simulink model "planLocalPathMPPI"  (R2024b)
settings: Solver=FixedStepAuto  StartTime=0.0  StopTime=inf  RelTol=1e-3  SampleTimeConstraint=STIndependent
StartFcn:
  | % clf
  | % rng(1,"twister");
  | % set_param([bdroot(gcb) '/TaskControllerIn/Simulink Signals/Confirm New Goal/newGoalBlock'],'Value','goalPose');
settings Model: Creator=cstabile  LastModifiedBy=apattass
settings DataIOCC: SaveOutput=off  SaveTime=off
settings OptimizationCC: BlockReduction=off  EnhancedBackFolding=on  PassReuseOutputArgsAs=Individual arguments  ZeroExternalMemoryAtStartup=off  ZeroInternalMemoryAtStartup=off  MaxStackSize=64  OptimizeBlockOrder=speed  DifferentSizesBufferReuse=on  OptimizationCustomize=off  EfficientTunableParamExpr=on
settings DebuggingCC: IntegerOverflowMsg=none  ParameterTunabilityLossMsg=error
settings ModelReferenceCC: UpdateModelReferenceTargets=IfOutOfDate
settings SFSimCC: SFSimEcho=off  SimTargetLang=C++
settings RTWCC: Description=Embedded Coder  SystemTargetFile=ert.tlc  TemplateMakefile=ert_default_tmf  Toolchain=Colcon Tools  GPUComputeCapability=3.5
settings CodeAppCC: ForceParamTrailComments=on  IgnoreCustomStorageClasses=off  OperatorAnnotations=on  SimulinkDataObjDesc=on  SFDataObjDesc=on  InsertBlockDesc=on
settings ERTTargetCC: InlinedParameterPlacement=Hierarchical  RootIOFormat=Structure reference  ERTCustomFileTemplate=example_file_process.tlc  DynamicArrayContainerType=coder::array

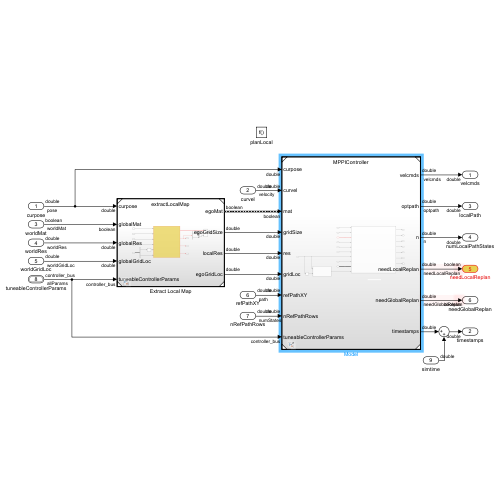
[thumbnail: Simulink's stored preview of the top-level diagram]
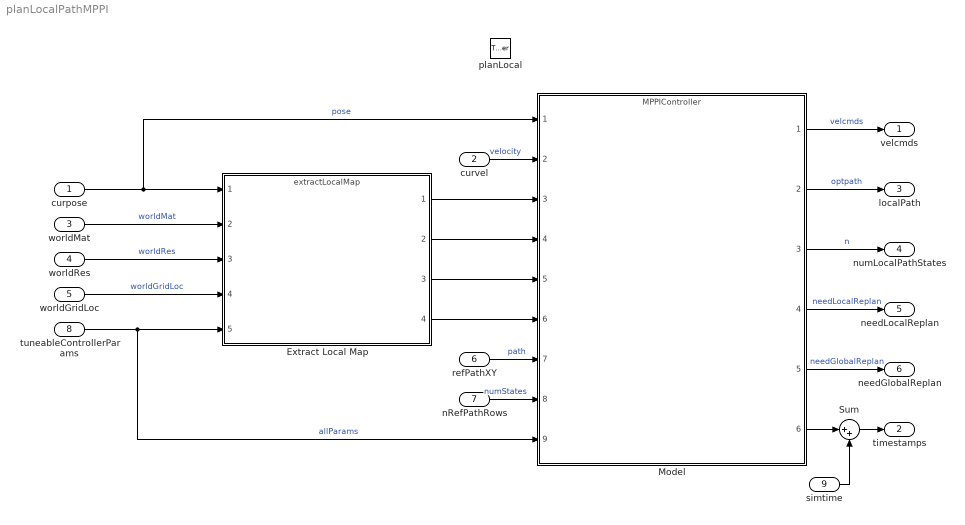
== system planLocalPathMPPI ==
  curpose : Inport  OutDataTypeStr=double  PortDimensions=3
  curvel : Inport  Port=2  OutDataTypeStr=double  PortDimensions=[1 2]
  worldMat : Inport  Port=3  OutDataTypeStr=boolean  PortDimensions=[1201 1201]
  worldRes : Inport  Port=4  OutDataTypeStr=double  PortDimensions=1
  worldGridLoc : Inport  Port=5  OutDataTypeStr=double  PortDimensions=2
  refPathXY : Inport  Port=6  OutDataTypeStr=double  PortDimensions=[10000 3]
  nRefPathRows : Inport  Port=7  OutDataTypeStr=double  PortDimensions=1
  tuneableControllerParams : Inport  Port=8  OutDataTypeStr=Bus: controller_bus  PortDimensions=1  BusOutputAsStruct=on
  simtime : Inport  Port=9  OutDataTypeStr=double  PortDimensions=1
  planLocal : TriggerPort  TriggerType=function-call  VariantControl=(inherit)  PortDimensions=1  TriggerSignalSampleTime=[0.10000000000000001,0]
  Extract Local Map : ModelReference  ModelNameDialog=extractLocalMap.slx  SimulationMode=Normal  ModelReferenceVersion=2.14
  Model : ModelReference  ModelNameDialog=MPPIController.slx  SimulationMode=Normal  ModelReferenceVersion=1.164
  Sum : Sum  Inputs=|++
  velcmds : Outport  OutDataTypeStr=double  PortDimensions=[1000 2]
  timestamps : Outport  Port=2  OutDataTypeStr=double  PortDimensions=[1000 1]
  localPath : Outport  Port=3  OutDataTypeStr=double  PortDimensions=[1000 3]
  numLocalPathStates : Outport  Port=4  OutDataTypeStr=double  PortDimensions=1
  needLocalReplan : Outport  Port=5  OutDataTypeStr=boolean  PortDimensions=1
  needGlobalReplan : Outport  Port=6  OutDataTypeStr=boolean  PortDimensions=1
  wires:
  curpose/1 -> Extract Local Map/1, Model/1  "pose"
  worldMat/1 -> Extract Local Map/2  "worldMat"
  tuneableControllerParams/1 -> Extract Local Map/5, Model/9  "allParams"
  worldRes/1 -> Extract Local Map/3  "worldRes"
  worldGridLoc/1 -> Extract Local Map/4  "worldGridLoc"
  nRefPathRows/1 -> Model/8  "numStates"
  Model/1 -> velcmds/1  "velcmds"
  Model/4 -> needLocalReplan/1  "needLocalReplan"
  Model/3 -> numLocalPathStates/1  "n"
  Model/2 -> localPath/1  "optpath"
  Model/5 -> needGlobalReplan/1  "needGlobalReplan"
  refPathXY/1 -> Model/7  "path"
  Extract Local Map/1 -> Model/3
  Extract Local Map/2 -> Model/4
  Extract Local Map/3 -> Model/5
  Extract Local Map/4 -> Model/6
  curvel/1 -> Model/2  "velocity"
  simtime/1 -> Sum/2
  Model/6 -> Sum/1
  Sum/1 -> timestamps/1
